simulink model "VRmodel2"  (R2021a)
settings: Solver=VariableStepAuto  StartTime=0.0  StopTime=800  RelTol=1e-3
undefined symbols (not defined in the file or in its folder): param
libraries: simulink x9, vrlib x1
settings Model: Creator=ania  LastModifiedBy=annasibilska-mroziewicz
settings SolverCC: AlgebraicLoopSolver=TrustRegion
settings DebuggingCC: SFMachineParentedDataDiag=warning
settings SFSimCC: CustomCodeUndefinedFunction=UseInterfaceOnly

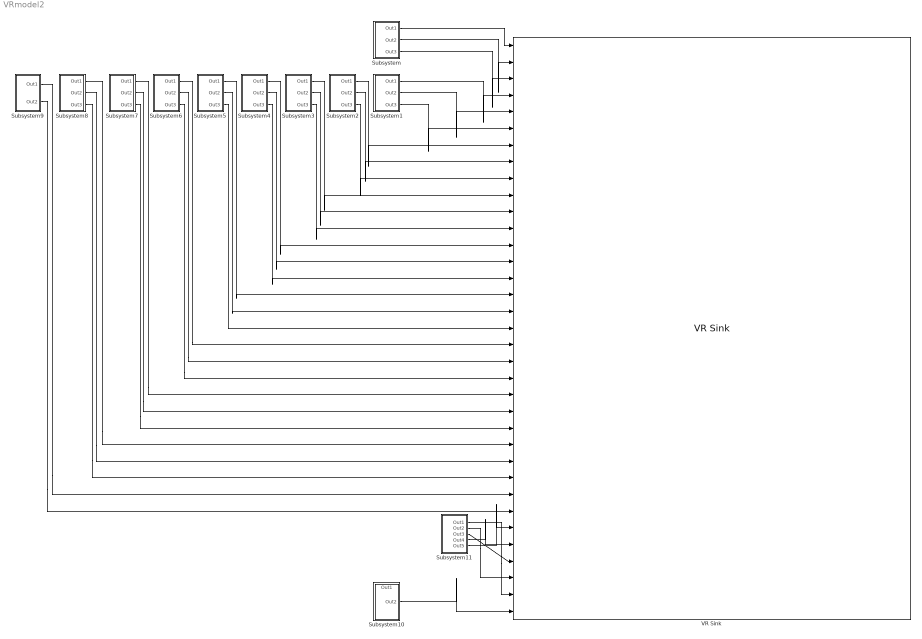
== system VRmodel2 ==
  Subsystem : Subsystem
  Subsystem1 : Subsystem
  Subsystem10 : Subsystem
      settings: PortSchema="{\"entries\":[{\"content\":{\"sides\":[{\"content\":{\"connectorIds\":[]},\"type\":\"ConnectorPlacement.EquallySpacedRectSide\",\"uuid\":\"3e4b479f-eebe-4db2-8806-dd619a093b4c\"},{\"content\":{\"connectorIds\":[\"Out1\"],\"side\":\"RIGHT\"},\"type\":\"ConnectorPlacement.EquallySpacedRectSide\",\"uuid\":\"cdaceeca-c530-403a-a620-8ccce5b6bd15\"},{\"content\":{\"connectorIds\":[\"Out2\"],\"side\":\"TOP\"},\"type\":\"ConnectorPlacement.EquallySpacedRectSide\",\"uuid\":\"eb53c295-fd49-4e3f-ac50-6d7a9d3182cb\"}]},\"type\":\"ConnectorPlacement.EquallySpacedConnector\",\"uuid\":\"b51d9349-5994-4002-abf8-8ec77c293e0f\"}],\"packageUris\":[\"http://schema.mathworks.com/mf0/Connector/R2020b\"],\"version\":\"1.0\"}"
  Subsystem11 : Subsystem
  Subsystem2 : Subsystem
  Subsystem3 : Subsystem
  Subsystem4 : Subsystem
  Subsystem5 : Subsystem
  Subsystem6 : Subsystem
  Subsystem7 : Subsystem
  Subsystem8 : Subsystem
  Subsystem9 : Subsystem
  VR Sink : vrlib/VR Sink  InstantiateOnLoad=on  SampleTime=0.1  ViewEnable=on  RemoteChange=off  RemoteView=off  FieldsWritten=człon1.rotation.4.1.1.double#człon1.translation.3.1.1.double#hea_Material.diffuseColor.3.1.1.double#czlon2.rotation.4.1.1.double#czlon2.translation.3.1.1.double#node_Material_0001.diffuseColor.3.1.1.double#czlon3.rotation.4.1.1.double#czlon3.translation.3.1.1.double#node_Material_0002.diffuseColor.3.1.1.double#czlon4.rotation.4.1.1.double#czlon4.translation.3.1.1.double#node_Material_0003.diffuseColor.3.1.1.double#czlon5.rotation.4.1.1.double#czlon5.translation.3.1.1.double#node_Material_0004.diffuseColor.3.1.1.double#czlon6.rotation.4.1.1.double#czlon6.translation.3.1.1.double#node_Material_0005.diffuseColor.3.1.1.double#czlon7.rotation.4.1.1.double#czlon7.translation.3.1.1.double#node_Material_0006.diffuseColor.3.1.1.double#czlon8.rotation.4.1.1.double#czlon8.translation.3.1.1.double#node_Material_0007.diffuseColor.3.1.1.double#czlon9.rotation.4.1.1.double#czlon9.translation.3.1.1.double#node_Material_0008.diffuseColor.3.1.1.double#czlon10.rotation.4.1.1.double#czlon10.translation.3.1.1.double#tracerP5.translation.3.1.1.double#tracerP4.translation.3.1.1.double#tracerP3.translation.3.1.1.double#tracerP2.translation.3.1.1.double#tracerP1.translation.3.1.1.double#points.point.3.-1.1.double  WorldFileName=snakeVR2.wrl  AutoView=off  VideoDimensions=[]  AllowVariableSize=off  FigureProperties="{'Position', 'Name', 'Viewpoint', 'CameraBound', 'CameraDirection', 'CameraPosition', 'CameraUpVector', 'ZoomFactor', 'Antialiasing', 'Headlight', 'Lighting', 'NavPanel', 'Sound', 'StatusBar', 'Stereo3D', 'Stereo3DCameraOffset', 'Stereo3DHIT', 'ToolBar', 'Textures', 'Transparency', 'Triad', 'Wireframe', 'NavZones', 'NavMode', 'NavSpeed', 'CaptureFileFormat', 'CaptureFileName', 'Record2DCompressMethod', 'Record2DCompressQuality', 'Record2D', 'Record2DFileName', 'Record2DFPS'; [1.0000000000000000e+00   5.0000000000000000e+01   1.4400000000000000e+03   7.9900000000000000e+02], '', 'bok', 'on', [0.0000000000000000e+00   0.0000000000000000e+00  -1.0000000000000000e+00], [0.0000000000000000e+00   0.0000000000000000e+00   0.0000000000000000e+00], [0.0000000000000000e+00   1.0000000000000000e+00   0.0000000000000000e+00], [1.0000000000000000e+00], 'on', 'on', 'on', 'halfbar', 'on', 'on', 'off', [1.0000000149011612e-01], [0.0000000000000000e+00], 'on', 'on', 'on', 'none', 'off', 'off', 'fly', 'normal', 'tif', '%f_anim_%n.tif', 'auto', [7.5000000000000000e+01], 'on', 'head_CC_4.avi', 'auto'}"
  wires:
  Subsystem/1(Out1) -> VR Sink/1
  Subsystem/2(Out2) -> VR Sink/2
  Subsystem/3(Out3) -> VR Sink/3
  Subsystem1/1(Out1) -> VR Sink/4
  Subsystem1/2(Out2) -> VR Sink/5
  Subsystem1/3(Out3) -> VR Sink/6
  Subsystem2/1(Out1) -> VR Sink/7
  Subsystem2/2(Out2) -> VR Sink/8
  Subsystem2/3(Out3) -> VR Sink/9
  Subsystem3/1(Out1) -> VR Sink/10
  Subsystem3/2(Out2) -> VR Sink/11
  Subsystem3/3(Out3) -> VR Sink/12
  Subsystem4/1(Out1) -> VR Sink/13
  Subsystem4/2(Out2) -> VR Sink/14
  Subsystem4/3(Out3) -> VR Sink/15
  Subsystem5/1(Out1) -> VR Sink/16
  Subsystem5/2(Out2) -> VR Sink/17
  Subsystem5/3(Out3) -> VR Sink/18
  Subsystem6/1(Out1) -> VR Sink/19
  Subsystem6/2(Out2) -> VR Sink/20
  Subsystem6/3(Out3) -> VR Sink/21
  Subsystem7/1(Out1) -> VR Sink/22
  Subsystem7/2(Out2) -> VR Sink/23
  Subsystem7/3(Out3) -> VR Sink/24
  Subsystem8/1(Out1) -> VR Sink/25
  Subsystem8/2(Out2) -> VR Sink/26
  Subsystem8/3(Out3) -> VR Sink/27
  Subsystem9/1(Out1) -> VR Sink/28
  Subsystem9/2(Out2) -> VR Sink/29
  Subsystem11/1(Out1) -> VR Sink/34
  Subsystem10/1(Out2) -> VR Sink/35
  Subsystem11/2(Out2) -> VR Sink/33
  Subsystem11/3(Out3) -> VR Sink/32
  Subsystem11/4(Out4) -> VR Sink/31
  Subsystem11/5(Out5) -> VR Sink/30

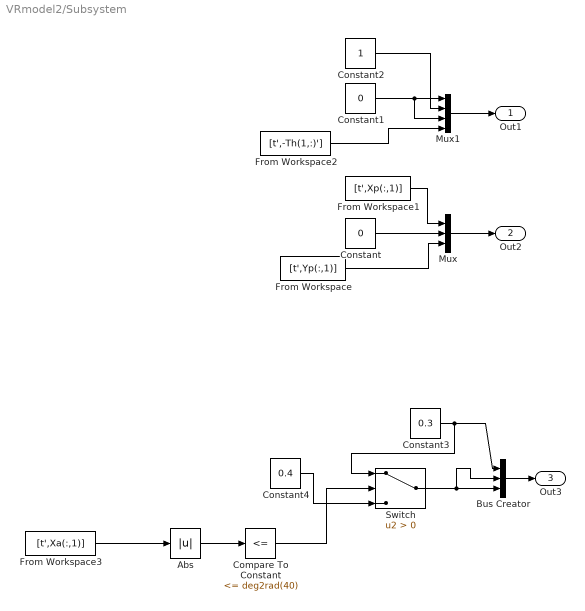
== system VRmodel2/Subsystem ==
  Abs : Abs
  Bus Creator : BusCreator  Inputs=3
  Compare To Constant : simulink/Logic and Bit Operations/Compare To Constant  relop=<=  const=deg2rad(40)  OutDataTypeStr=boolean
  Constant : Constant  Value=0
  Constant1 : Constant  Value=0
  Constant2 : Constant
  Constant3 : Constant  Value=0.3
  Constant4 : Constant  Value=0.4
  From Workspace : FromWorkspace  VariableName=[t',Yp(:,1)]
  From Workspace1 : FromWorkspace  VariableName=[t',Xp(:,1)]
  From Workspace2 : FromWorkspace  VariableName=[t',-Th(1,:)']
  From Workspace3 : FromWorkspace  VariableName=[t',Xa(:,1)]
  Mux : Mux  Inputs=3
  Mux1 : Mux
  Switch : Switch  Criteria=u2 > Threshold
  Out1 : Outport  VectorParamsAs1DForOutWhenUnconnected=off
  Out2 : Outport  Port=2  VectorParamsAs1DForOutWhenUnconnected=off
  Out3 : Outport  Port=3  VectorParamsAs1DForOutWhenUnconnected=off
  wires:
  Mux1/1 -> Out1/1
  Mux/1 -> Out2/1
  Constant/1 -> Mux/2
  Constant1/1 -> Mux1/1, Mux1/3
  From Workspace/1 -> Mux/3
  From Workspace1/1 -> Mux/1
  Switch/1 -> Bus Creator/2, Bus Creator/3
  Constant3/1 -> Switch/1, Bus Creator/1
  Constant4/1 -> Switch/3
  Bus Creator/1 -> Out3/1
  From Workspace3/1 -> Abs/1
  Compare To Constant/1 -> Switch/2
  Abs/1 -> Compare To Constant/1
  From Workspace2/1 -> Mux1/4
  Constant2/1 -> Mux1/2

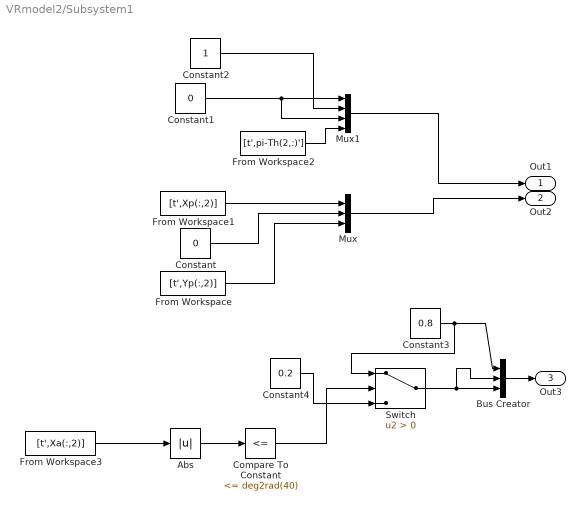
== system VRmodel2/Subsystem1 ==
  Abs : Abs
  Bus Creator : BusCreator  Inputs=3
  Compare To Constant : simulink/Logic and Bit Operations/Compare To Constant  relop=<=  const=deg2rad(40)  OutDataTypeStr=boolean
  Constant : Constant  Value=0
  Constant1 : Constant  Value=0
  Constant2 : Constant
  Constant3 : Constant  Value=0.8
  Constant4 : Constant  Value=0.2
  From Workspace : FromWorkspace  VariableName=[t',Yp(:,2)]
  From Workspace1 : FromWorkspace  VariableName=[t',Xp(:,2)]
  From Workspace2 : FromWorkspace  VariableName=[t',pi-Th(2,:)']
  From Workspace3 : FromWorkspace  VariableName=[t',Xa(:,2)]
  Mux : Mux  Inputs=3
  Mux1 : Mux
  Switch : Switch  Criteria=u2 > Threshold
  Out1 : Outport  VectorParamsAs1DForOutWhenUnconnected=off
  Out2 : Outport  Port=2  VectorParamsAs1DForOutWhenUnconnected=off
  Out3 : Outport  Port=3  VectorParamsAs1DForOutWhenUnconnected=off
  wires:
  Mux1/1 -> Out1/1
  Constant2/1 -> Mux1/2
  Mux/1 -> Out2/1
  Constant/1 -> Mux/2
  From Workspace2/1 -> Mux1/4
  Constant1/1 -> Mux1/1, Mux1/3
  From Workspace1/1 -> Mux/1
  From Workspace/1 -> Mux/3
  Bus Creator/1 -> Out3/1
  Constant3/1 -> Switch/1, Bus Creator/1
  Switch/1 -> Bus Creator/2, Bus Creator/3
  Compare To Constant/1 -> Switch/2
  Constant4/1 -> Switch/3
  From Workspace3/1 -> Abs/1
  Abs/1 -> Compare To Constant/1

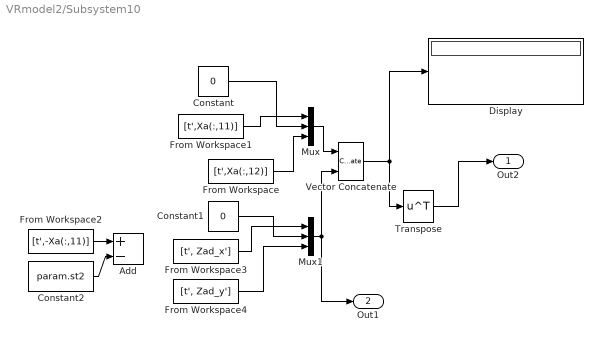
== system VRmodel2/Subsystem10 ==
  Add : Sum  Inputs=+-
  Constant : Constant  Value=0
  Constant1 : Constant  Value=0
  Constant2 : Constant  Value=param.st2
  Display : Display
  From Workspace : FromWorkspace  VariableName=[t',Xa(:,12)]
  From Workspace1 : FromWorkspace  VariableName=[t',Xa(:,11)]
  From Workspace2 : FromWorkspace  VariableName=[t',-Xa(:,11)]
  From Workspace3 : FromWorkspace  VariableName=[t', Zad_x']
  From Workspace4 : FromWorkspace  VariableName=[t', Zad_y']
  Mux : Mux  Inputs=3
  Mux1 : Mux  Inputs=3
  Transpose : Math  Operator=transpose  SaturateOnIntegerOverflow=on
  Vector Concatenate : Concatenate  Mode=Multidimensional array  ConcatenateDimension=2
  Out2 : Outport  VectorParamsAs1DForOutWhenUnconnected=off
  Out1 : Outport  Port=2  VectorParamsAs1DForOutWhenUnconnected=off
  wires:
  Mux/1 -> Vector Concatenate/1
  From Workspace/1 -> Mux/3
  Vector Concatenate/1 -> Transpose/1, Display/1
  Constant/1 -> Mux/2
  Mux1/1 -> Vector Concatenate/2, Out1/1
  Constant1/1 -> Mux1/2
  From Workspace2/1 -> Add/1
  Constant2/1 -> Add/2
  From Workspace4/1 -> Mux1/3
  Transpose/1 -> Out2/1
  From Workspace3/1 -> Mux1/1
  From Workspace1/1 -> Mux/1

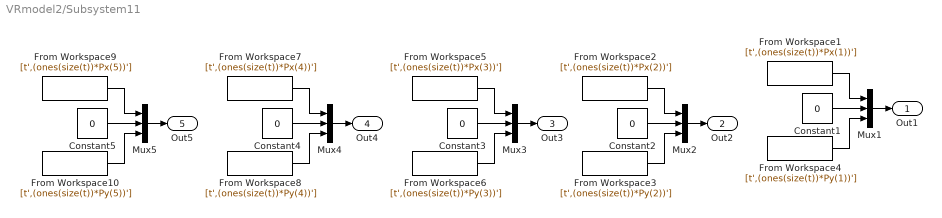
== system VRmodel2/Subsystem11 ==
  Constant{1..5} (5 alike) : Constant  Value=0
  From Workspace1 : FromWorkspace  VariableName=[t',(ones(size(t))*Px(1))']
  From Workspace10 : FromWorkspace  VariableName=[t',(ones(size(t))*Py(5))']
  From Workspace2 : FromWorkspace  VariableName=[t',(ones(size(t))*Px(2))']
  From Workspace3 : FromWorkspace  VariableName=[t',(ones(size(t))*Py(2))']
  From Workspace4 : FromWorkspace  VariableName=[t',(ones(size(t))*Py(1))']
  From Workspace5 : FromWorkspace  VariableName=[t',(ones(size(t))*Px(3))']
  From Workspace6 : FromWorkspace  VariableName=[t',(ones(size(t))*Py(3))']
  From Workspace7 : FromWorkspace  VariableName=[t',(ones(size(t))*Px(4))']
  From Workspace8 : FromWorkspace  VariableName=[t',(ones(size(t))*Py(4))']
  From Workspace9 : FromWorkspace  VariableName=[t',(ones(size(t))*Px(5))']
  Mux{1..5} (5 alike) : Mux  Inputs=3
  Out1 : Outport
  Out2 : Outport  Port=2
  Out3 : Outport  Port=3
  Out4 : Outport  Port=4
  Out5 : Outport  Port=5
  wires:
  Constant1/1 -> Mux1/2
  Mux1/1 -> Out1/1
  From Workspace4/1 -> Mux1/3
  From Workspace1/1 -> Mux1/1
  Constant2/1 -> Mux2/2
  From Workspace3/1 -> Mux2/3
  Mux2/1 -> Out2/1
  From Workspace2/1 -> Mux2/1
  Constant3/1 -> Mux3/2
  From Workspace6/1 -> Mux3/3
  Mux3/1 -> Out3/1
  From Workspace5/1 -> Mux3/1
  Constant4/1 -> Mux4/2
  From Workspace8/1 -> Mux4/3
  Mux4/1 -> Out4/1
  From Workspace7/1 -> Mux4/1
  Constant5/1 -> Mux5/2
  From Workspace10/1 -> Mux5/3
  Mux5/1 -> Out5/1
  From Workspace9/1 -> Mux5/1

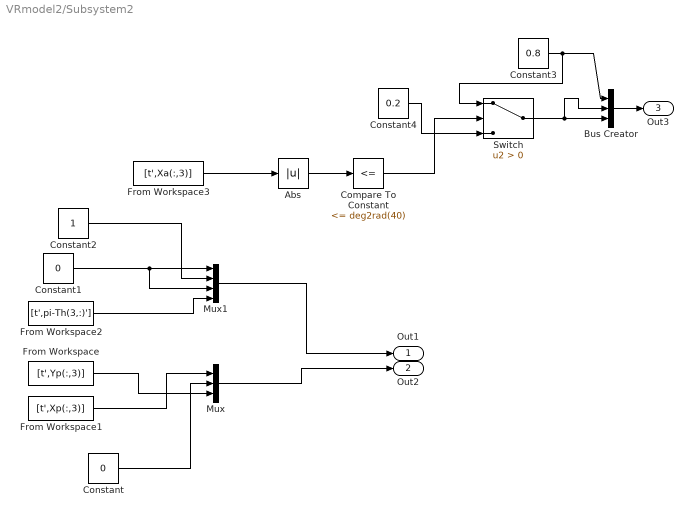
== system VRmodel2/Subsystem2 ==
  Abs : Abs
  Bus Creator : BusCreator  Inputs=3
  Compare To Constant : simulink/Logic and Bit Operations/Compare To Constant  relop=<=  const=deg2rad(40)  OutDataTypeStr=boolean
  Constant : Constant  Value=0
  Constant1 : Constant  Value=0
  Constant2 : Constant
  Constant3 : Constant  Value=0.8
  Constant4 : Constant  Value=0.2
  From Workspace : FromWorkspace  VariableName=[t',Yp(:,3)]
  From Workspace1 : FromWorkspace  VariableName=[t',Xp(:,3)]
  From Workspace2 : FromWorkspace  VariableName=[t',pi-Th(3,:)']
  From Workspace3 : FromWorkspace  VariableName=[t',Xa(:,3)]
  Mux : Mux  Inputs=3
  Mux1 : Mux
  Switch : Switch  Criteria=u2 > Threshold
  Out1 : Outport  VectorParamsAs1DForOutWhenUnconnected=off
  Out2 : Outport  Port=2  VectorParamsAs1DForOutWhenUnconnected=off
  Out3 : Outport  Port=3  VectorParamsAs1DForOutWhenUnconnected=off
  wires:
  Mux1/1 -> Out1/1
  Constant2/1 -> Mux1/2
  Mux/1 -> Out2/1
  Constant/1 -> Mux/2
  From Workspace2/1 -> Mux1/4
  Constant1/1 -> Mux1/1, Mux1/3
  From Workspace1/1 -> Mux/1
  From Workspace/1 -> Mux/3
  Bus Creator/1 -> Out3/1
  Constant3/1 -> Switch/1, Bus Creator/1
  Switch/1 -> Bus Creator/2, Bus Creator/3
  Compare To Constant/1 -> Switch/2
  Constant4/1 -> Switch/3
  From Workspace3/1 -> Abs/1
  Abs/1 -> Compare To Constant/1

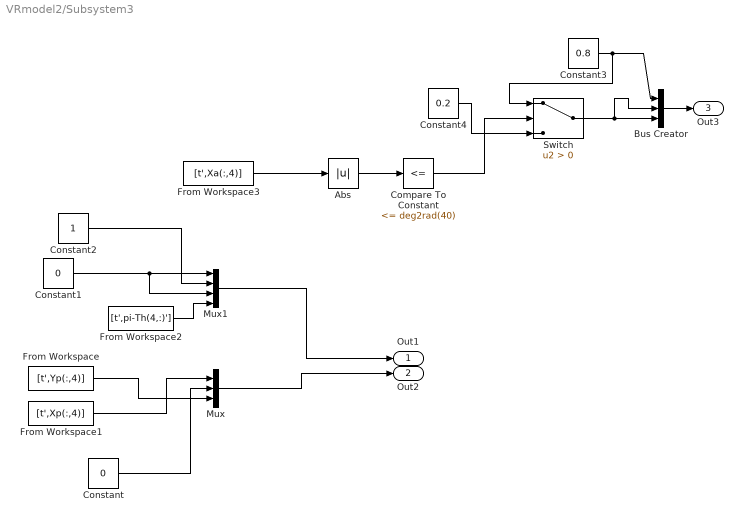
== system VRmodel2/Subsystem3 ==
  Abs : Abs
  Bus Creator : BusCreator  Inputs=3
  Compare To Constant : simulink/Logic and Bit Operations/Compare To Constant  relop=<=  const=deg2rad(40)  OutDataTypeStr=boolean
  Constant : Constant  Value=0
  Constant1 : Constant  Value=0
  Constant2 : Constant
  Constant3 : Constant  Value=0.8
  Constant4 : Constant  Value=0.2
  From Workspace : FromWorkspace  VariableName=[t',Yp(:,4)]
  From Workspace1 : FromWorkspace  VariableName=[t',Xp(:,4)]
  From Workspace2 : FromWorkspace  VariableName=[t',pi-Th(4,:)']
  From Workspace3 : FromWorkspace  VariableName=[t',Xa(:,4)]
  Mux : Mux  Inputs=3
  Mux1 : Mux
  Switch : Switch  Criteria=u2 > Threshold
  Out1 : Outport  VectorParamsAs1DForOutWhenUnconnected=off
  Out2 : Outport  Port=2  VectorParamsAs1DForOutWhenUnconnected=off
  Out3 : Outport  Port=3  VectorParamsAs1DForOutWhenUnconnected=off
  wires:
  Mux1/1 -> Out1/1
  Constant2/1 -> Mux1/2
  Mux/1 -> Out2/1
  Constant/1 -> Mux/2
  From Workspace2/1 -> Mux1/4
  Constant1/1 -> Mux1/1, Mux1/3
  From Workspace1/1 -> Mux/1
  From Workspace/1 -> Mux/3
  Bus Creator/1 -> Out3/1
  Constant3/1 -> Switch/1, Bus Creator/1
  Switch/1 -> Bus Creator/2, Bus Creator/3
  Compare To Constant/1 -> Switch/2
  Constant4/1 -> Switch/3
  From Workspace3/1 -> Abs/1
  Abs/1 -> Compare To Constant/1

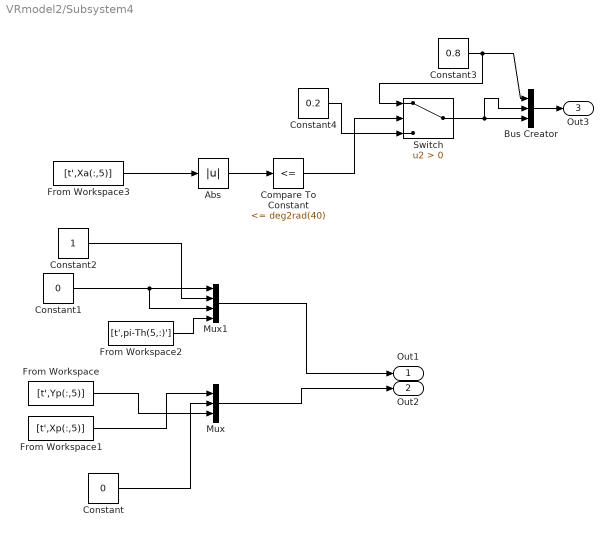
== system VRmodel2/Subsystem4 ==
  Abs : Abs
  Bus Creator : BusCreator  Inputs=3
  Compare To Constant : simulink/Logic and Bit Operations/Compare To Constant  relop=<=  const=deg2rad(40)  OutDataTypeStr=boolean
  Constant : Constant  Value=0
  Constant1 : Constant  Value=0
  Constant2 : Constant
  Constant3 : Constant  Value=0.8
  Constant4 : Constant  Value=0.2
  From Workspace : FromWorkspace  VariableName=[t',Yp(:,5)]
  From Workspace1 : FromWorkspace  VariableName=[t',Xp(:,5)]
  From Workspace2 : FromWorkspace  VariableName=[t',pi-Th(5,:)']
  From Workspace3 : FromWorkspace  VariableName=[t',Xa(:,5)]
  Mux : Mux  Inputs=3
  Mux1 : Mux
  Switch : Switch  Criteria=u2 > Threshold
  Out1 : Outport  VectorParamsAs1DForOutWhenUnconnected=off
  Out2 : Outport  Port=2  VectorParamsAs1DForOutWhenUnconnected=off
  Out3 : Outport  Port=3  VectorParamsAs1DForOutWhenUnconnected=off
  wires:
  Mux1/1 -> Out1/1
  Constant2/1 -> Mux1/2
  Mux/1 -> Out2/1
  Constant/1 -> Mux/2
  From Workspace2/1 -> Mux1/4
  Constant1/1 -> Mux1/1, Mux1/3
  From Workspace1/1 -> Mux/1
  From Workspace/1 -> Mux/3
  Bus Creator/1 -> Out3/1
  Constant3/1 -> Switch/1, Bus Creator/1
  Switch/1 -> Bus Creator/2, Bus Creator/3
  Compare To Constant/1 -> Switch/2
  Constant4/1 -> Switch/3
  From Workspace3/1 -> Abs/1
  Abs/1 -> Compare To Constant/1

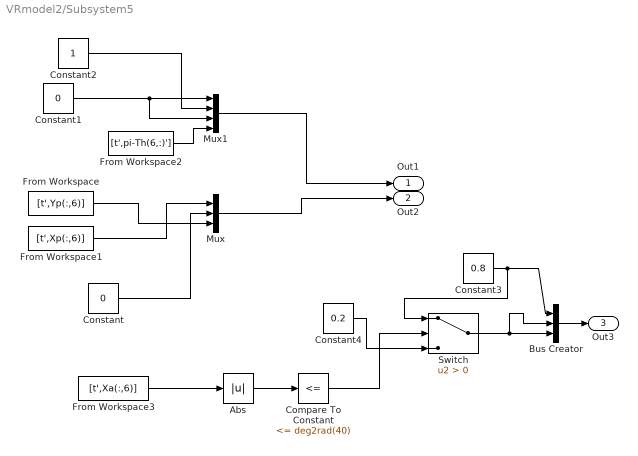
== system VRmodel2/Subsystem5 ==
  Abs : Abs
  Bus Creator : BusCreator  Inputs=3
  Compare To Constant : simulink/Logic and Bit Operations/Compare To Constant  relop=<=  const=deg2rad(40)  OutDataTypeStr=boolean
  Constant : Constant  Value=0
  Constant1 : Constant  Value=0
  Constant2 : Constant
  Constant3 : Constant  Value=0.8
  Constant4 : Constant  Value=0.2
  From Workspace : FromWorkspace  VariableName=[t',Yp(:,6)]
  From Workspace1 : FromWorkspace  VariableName=[t',Xp(:,6)]
  From Workspace2 : FromWorkspace  VariableName=[t',pi-Th(6,:)']
  From Workspace3 : FromWorkspace  VariableName=[t',Xa(:,6)]
  Mux : Mux  Inputs=3
  Mux1 : Mux
  Switch : Switch  Criteria=u2 > Threshold
  Out1 : Outport  VectorParamsAs1DForOutWhenUnconnected=off
  Out2 : Outport  Port=2  VectorParamsAs1DForOutWhenUnconnected=off
  Out3 : Outport  Port=3  VectorParamsAs1DForOutWhenUnconnected=off
  wires:
  Mux1/1 -> Out1/1
  Constant2/1 -> Mux1/2
  Mux/1 -> Out2/1
  Constant/1 -> Mux/2
  From Workspace2/1 -> Mux1/4
  Constant1/1 -> Mux1/1, Mux1/3
  From Workspace1/1 -> Mux/1
  From Workspace/1 -> Mux/3
  Bus Creator/1 -> Out3/1
  Constant3/1 -> Switch/1, Bus Creator/1
  Switch/1 -> Bus Creator/2, Bus Creator/3
  Compare To Constant/1 -> Switch/2
  Constant4/1 -> Switch/3
  From Workspace3/1 -> Abs/1
  Abs/1 -> Compare To Constant/1

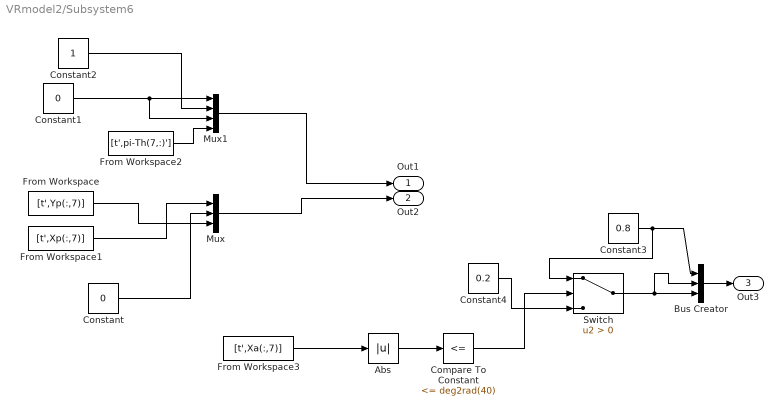
== system VRmodel2/Subsystem6 ==
  Abs : Abs
  Bus Creator : BusCreator  Inputs=3
  Compare To Constant : simulink/Logic and Bit Operations/Compare To Constant  relop=<=  const=deg2rad(40)  OutDataTypeStr=boolean
  Constant : Constant  Value=0
  Constant1 : Constant  Value=0
  Constant2 : Constant
  Constant3 : Constant  Value=0.8
  Constant4 : Constant  Value=0.2
  From Workspace : FromWorkspace  VariableName=[t',Yp(:,7)]
  From Workspace1 : FromWorkspace  VariableName=[t',Xp(:,7)]
  From Workspace2 : FromWorkspace  VariableName=[t',pi-Th(7,:)']
  From Workspace3 : FromWorkspace  VariableName=[t',Xa(:,7)]
  Mux : Mux  Inputs=3
  Mux1 : Mux
  Switch : Switch  Criteria=u2 > Threshold
  Out1 : Outport  VectorParamsAs1DForOutWhenUnconnected=off
  Out2 : Outport  Port=2  VectorParamsAs1DForOutWhenUnconnected=off
  Out3 : Outport  Port=3  VectorParamsAs1DForOutWhenUnconnected=off
  wires:
  Mux1/1 -> Out1/1
  Constant2/1 -> Mux1/2
  Mux/1 -> Out2/1
  Constant/1 -> Mux/2
  From Workspace2/1 -> Mux1/4
  Constant1/1 -> Mux1/1, Mux1/3
  From Workspace1/1 -> Mux/1
  From Workspace/1 -> Mux/3
  Bus Creator/1 -> Out3/1
  Constant3/1 -> Switch/1, Bus Creator/1
  Switch/1 -> Bus Creator/2, Bus Creator/3
  Compare To Constant/1 -> Switch/2
  Constant4/1 -> Switch/3
  From Workspace3/1 -> Abs/1
  Abs/1 -> Compare To Constant/1

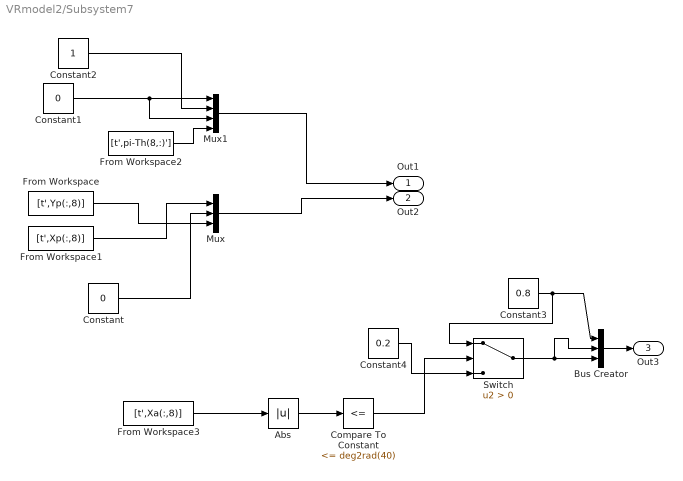
== system VRmodel2/Subsystem7 ==
  Abs : Abs
  Bus Creator : BusCreator  Inputs=3
  Compare To Constant : simulink/Logic and Bit Operations/Compare To Constant  relop=<=  const=deg2rad(40)  OutDataTypeStr=boolean
  Constant : Constant  Value=0
  Constant1 : Constant  Value=0
  Constant2 : Constant
  Constant3 : Constant  Value=0.8
  Constant4 : Constant  Value=0.2
  From Workspace : FromWorkspace  VariableName=[t',Yp(:,8)]
  From Workspace1 : FromWorkspace  VariableName=[t',Xp(:,8)]
  From Workspace2 : FromWorkspace  VariableName=[t',pi-Th(8,:)']
  From Workspace3 : FromWorkspace  VariableName=[t',Xa(:,8)]
  Mux : Mux  Inputs=3
  Mux1 : Mux
  Switch : Switch  Criteria=u2 > Threshold
  Out1 : Outport  VectorParamsAs1DForOutWhenUnconnected=off
  Out2 : Outport  Port=2  VectorParamsAs1DForOutWhenUnconnected=off
  Out3 : Outport  Port=3  VectorParamsAs1DForOutWhenUnconnected=off
  wires:
  Mux1/1 -> Out1/1
  Constant2/1 -> Mux1/2
  Mux/1 -> Out2/1
  Constant/1 -> Mux/2
  From Workspace2/1 -> Mux1/4
  Constant1/1 -> Mux1/1, Mux1/3
  From Workspace1/1 -> Mux/1
  From Workspace/1 -> Mux/3
  Bus Creator/1 -> Out3/1
  Constant3/1 -> Switch/1, Bus Creator/1
  Switch/1 -> Bus Creator/2, Bus Creator/3
  Compare To Constant/1 -> Switch/2
  Constant4/1 -> Switch/3
  From Workspace3/1 -> Abs/1
  Abs/1 -> Compare To Constant/1

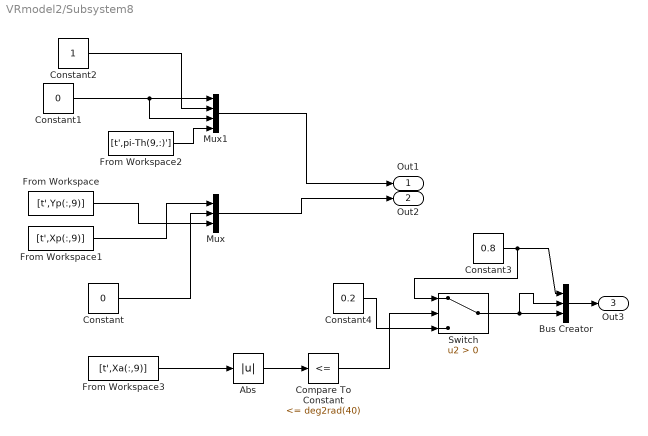
== system VRmodel2/Subsystem8 ==
  Abs : Abs
  Bus Creator : BusCreator  Inputs=3
  Compare To Constant : simulink/Logic and Bit Operations/Compare To Constant  relop=<=  const=deg2rad(40)  OutDataTypeStr=boolean
  Constant : Constant  Value=0
  Constant1 : Constant  Value=0
  Constant2 : Constant
  Constant3 : Constant  Value=0.8
  Constant4 : Constant  Value=0.2
  From Workspace : FromWorkspace  VariableName=[t',Yp(:,9)]
  From Workspace1 : FromWorkspace  VariableName=[t',Xp(:,9)]
  From Workspace2 : FromWorkspace  VariableName=[t',pi-Th(9,:)']
  From Workspace3 : FromWorkspace  VariableName=[t',Xa(:,9)]
  Mux : Mux  Inputs=3
  Mux1 : Mux
  Switch : Switch  Criteria=u2 > Threshold
  Out1 : Outport  VectorParamsAs1DForOutWhenUnconnected=off
  Out2 : Outport  Port=2  VectorParamsAs1DForOutWhenUnconnected=off
  Out3 : Outport  Port=3  VectorParamsAs1DForOutWhenUnconnected=off
  wires:
  Mux1/1 -> Out1/1
  Constant2/1 -> Mux1/2
  Mux/1 -> Out2/1
  Constant/1 -> Mux/2
  From Workspace2/1 -> Mux1/4
  Constant1/1 -> Mux1/1, Mux1/3
  From Workspace1/1 -> Mux/1
  From Workspace/1 -> Mux/3
  Bus Creator/1 -> Out3/1
  Constant3/1 -> Switch/1, Bus Creator/1
  Switch/1 -> Bus Creator/2, Bus Creator/3
  Compare To Constant/1 -> Switch/2
  Constant4/1 -> Switch/3
  From Workspace3/1 -> Abs/1
  Abs/1 -> Compare To Constant/1

== system VRmodel2/Subsystem9 ==
  Constant : Constant  Value=0
  Constant1 : Constant  Value=0
  Constant2 : Constant
  From Workspace : FromWorkspace  VariableName=[t',Yp(:,10)]
  From Workspace1 : FromWorkspace  VariableName=[t',Xp(:,10)]
  From Workspace2 : FromWorkspace  VariableName=[t',-Th(10,:)']
  Mux : Mux  Inputs=3
  Mux1 : Mux
  Out1 : Outport  VectorParamsAs1DForOutWhenUnconnected=off
  Out2 : Outport  Port=2  VectorParamsAs1DForOutWhenUnconnected=off
  wires:
  Mux1/1 -> Out1/1
  Constant2/1 -> Mux1/2
  Mux/1 -> Out2/1
  Constant/1 -> Mux/2
  From Workspace2/1 -> Mux1/4
  Constant1/1 -> Mux1/1, Mux1/3
  From Workspace1/1 -> Mux/1
  From Workspace/1 -> Mux/3
